simulink model "telemedicine_screening_workflow"  (R2026a)
settings: Solver=VariableStepAuto
settings Model: Creator=hk3202  LastModifiedBy=hk3202

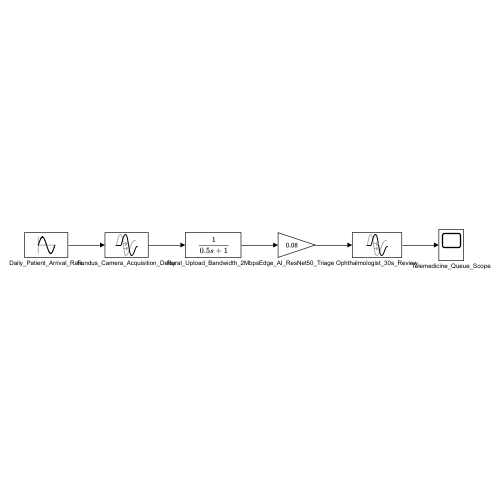
[thumbnail: Simulink's stored preview of the top-level diagram]
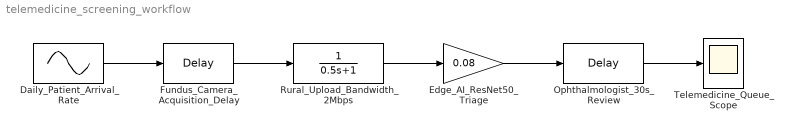
== system telemedicine_screening_workflow ==
  Daily_Patient_Arrival_Rate : Sin  Amplitude=50  Bias=333  Frequency=2*pi/24  SampleTime=0
  Edge_AI_ResNet50_Triage : Gain  Gain=0.08
  Fundus_Camera_Acquisition_Delay : TransportDelay  DelayTime=3.0
  Ophthalmologist_30s_Review : TransportDelay  DelayTime=0.5
  Rural_Upload_Bandwidth_2Mbps : TransferFcn  Denominator=[0.5 1]
  Telemedicine_Queue_Scope : Scope
  wires:
  Daily_Patient_Arrival_Rate/1 -> Fundus_Camera_Acquisition_Delay/1
  Fundus_Camera_Acquisition_Delay/1 -> Rural_Upload_Bandwidth_2Mbps/1
  Rural_Upload_Bandwidth_2Mbps/1 -> Edge_AI_ResNet50_Triage/1
  Edge_AI_ResNet50_Triage/1 -> Ophthalmologist_30s_Review/1
  Ophthalmologist_30s_Review/1 -> Telemedicine_Queue_Scope/1
